simulink model "MPU9250"  (R2020b)
settings: Solver=FixedStepAuto  StartTime=0.0  StopTime=inf  FixedStep=1/500  RelTol=1e-3
libraries: sm_lib x4, nesl_utility x4, mspfiltlib x1, arduinosensorlib x1
settings Model: SILPILModeSetting=veronly  ExtModeTrigDuration=2  Creator=Tommaso  LastModifiedBy=Tommaso
settings OptimizationCC: EnhancedBackFolding=on  PassReuseOutputArgsAs=Individual arguments  ZeroExternalMemoryAtStartup=off  ZeroInternalMemoryAtStartup=off  MaxStackSize=64  OptimizeBlockOrder=speed  DifferentSizesBufferReuse=on  OptimizationCustomize=off  EfficientTunableParamExpr=on
settings DebuggingCC: ParameterTunabilityLossMsg=error
settings HardwareCC: ProdBitPerInt=16  ProdBitPerPointer=16  ProdBitPerSizeT=16  ProdBitPerPtrDiffT=16  ProdLargestAtomicFloat=None  ProdWordSize=8  ProdHWDeviceType=Atmel->AVR  UseEmbeddedCoderFeatures=off  UseSimulinkCoderFeatures=off
settings SFSimCC: MATLABDynamicMemAlloc=off
settings RTWCC: Description=Embedded Coder  SystemTargetFile=ert.tlc  HardwareBoard=Arduino Uno  TemplateMakefile=ert_default_tmf  Toolchain=Arduino AVR
settings CodeAppCC: ForceParamTrailComments=on  IgnoreCustomStorageClasses=off  OperatorAnnotations=on  SimulinkDataObjDesc=on  SFDataObjDesc=on  InsertBlockDesc=on
settings ERTTargetCC: SupportContinuousTime=on  SupportNonInlinedSFcns=on  SupportVariableSizeSignals=on  ExtModeStaticAllocSize=250
settings ExplorerConfigSet: InternalSimMechanicsExplorerSettings="<ExplorerConfiguration><canonicalview>aerospace</canonicalview><AnimationSetting><BasePlaybackSpeed>1.0</BasePlaybackSpeed><PlaybackSpeedFactor>1.0</PlaybackSpeedFactor></AnimationSetting><TilePanel><TileInfo><Tiles Columns=\"1\" Count=\"1\" Rows=\"1\"><Column Weight=\"1\"/><Row Weight=\"1\"/><Tile Height=\"1\" Width=\"1\" X=\"0\" Y=\"0\"/></Tiles></TileInfo><SceneInfo><SceneViewer><BGColor><R>1</R><G>1</G><B>1</B></BGColor><Camera><DoPerspective>off</DoPerspective><Position><X>-0.693082754697760484</X><Y>0.369421598530021988</Y><Z>-0.361362961081841516</Z></Position><Center><X>0.12253292156436324</X><Y>-0.0789962126630676664</Y><Z>0.00427693723400418557</Z></Center><Up><X>0.320163956155274265</X><Y>-0.176600674730688856</Y><Z>-0.930756274684016782</Z></Up><ViewLimDist>1</ViewLimDist><YLim>0.1588242526875695</YLim><XLim>0.267697134651695201</XLim></Camera></SceneViewer></SceneInfo></TilePanel><MechEditorPanel><Cameras/><GfxPanelCameraMap/><VideoCreator><PlaybackSpeedRatio>1.0</PlaybackSpeedRatio><FrameRate>30</FrameRate><VideoFormat>Motion JPEG AVI</VideoFormat><FrameSize>auto</FrameSize></VideoCreator></MechEditorPanel></ExplorerConfiguration>"

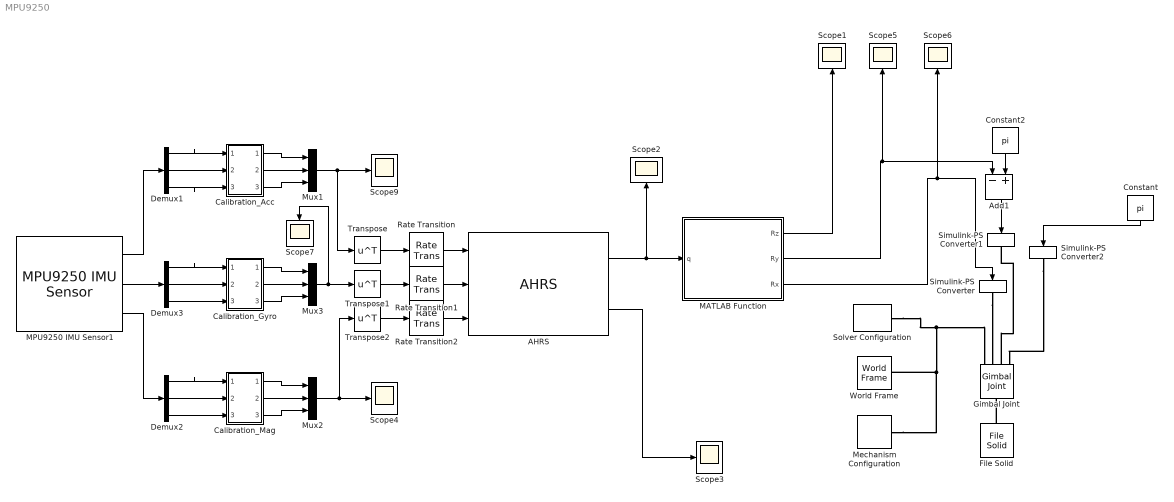
== system MPU9250 ==
  AHRS : mspfiltlib/AHRS  DispRefFrame=NED  DecimationFactor=1  InitialProcessNoise=ahrsfilter.defaultProcessNoise  OrientationFormat=quaternion  SimulateUsing=Interpreted execution  AccelerometerNoise=0.05  GyroscopeNoise=1  MagnetometerNoise=3  GyroscopeDriftNoise=3.0462e-3  LinearAccelerationNoise=0.01  MagneticDisturbanceNoise=0.5  LinearAccelerationDecayFactor=0.14  MagneticDisturbanceDecayFactor=0.08  ExpectedMagneticFieldStrength=40
      settings: SourceProductBaseCode=TF,NV
  Add1 : Sum  Inputs=-+
  Calibration_Acc : Subsystem
  Calibration_Gyro : Subsystem
  Calibration_Mag : Subsystem
  Constant : Constant  Value=pi
  Constant2 : Constant  Value=pi
  Demux1 : Demux  Outputs=3
  Demux2 : Demux  Outputs=3
  Demux3 : Demux  Outputs=3
  File Solid : sm_lib/Body Elements/File Solid  ExtGeomFileName=C:\Users\Tommaso\università\Controlli Automatici\Progetto\Solidworks\Drone.stl  UnitType=Custom  ExtGeomFileUnits=mm  StepReaderType=HEX  ExportConvexHullGeometry=off  InertiaType=Custom  Mass=1  MassUnits=kg  CenterOfMass=[150 150 40]  CenterOfMassUnits=mm  MomentsOfInertia=[1 1 1]  MomentsOfInertiaUnits=kg*m^2  ProductsOfInertia=[0 0 0]  ProductsOfInertiaUnits=kg*m^2  BasedOnType=DensityFromFile  Density=1000  DensityUnits=kg/m^3  DoExposeReferenceFrame=off  SerializedFrames=<Frames><Frame><Id>Frame1</Id><Value><Name>F1</Name><Origin><Source>CenterOfMassFrame</Source><FeatureName></FeatureName></Origin><PrimaryAxis><DefinedDirection>+Z</DefinedDirection><Source>ReferenceFrame</Source><SourceDirection>-Z</SourceDirection><FeatureName></FeatureName></PrimaryAxis><SecondaryAxis><DefinedDirection>+X</DefinedDirection><Source>ReferenceFrame</Source><SourceDirection>-X</SourceDirection><FeatureName></FeatureName></SecondaryAxis></Value></Frame></Frames>  GraphicType=FromGeometry  MarkerShape=Sphere  MarkerSize=10  GraphicVisPropType=SimpleVisualProperties  GraphicDiffuseColor=[0.6 0.6 0.6]  GraphicSpecularColor=[0.5 0.5 0.5 1.0]  GraphicAmbientColor=[0.15 0.15 0.15 1.0]  GraphicEmissiveColor=[0.0 0.0 0.0 1.0]  GraphicShininess=75  GraphicOpacity=1.0
  Gimbal Joint : sm_lib/Joints/Gimbal Joint  JointMode=Normal  SenseConstraintForce=off  SenseConstraintForceX=off  SenseConstraintForceY=off  SenseConstraintForceZ=off  SenseConstraintTorque=off  SenseConstraintTorqueX=off  SenseConstraintTorqueY=off  SenseConstraintTorqueZ=off  SenseTotalForce=off  SenseTotalForceX=off  SenseTotalForceY=off  SenseTotalForceZ=off  SenseTotalTorque=off  SenseTotalTorqueX=off  SenseTotalTorqueY=off  SenseTotalTorqueZ=off  CompositeWrenchDir=FollowerOnBase  CompositeWrenchFrame=BaseFrame  RxEquilibriumPosition=0  RxEquilibriumPositionUnits=deg  RxSpringStiffness=0  RxSpringStiffnessUnits=N*m/deg  RxDampingCoefficient=0  RxDampingCoefficientUnits=N*m/(deg/s)  RxTorqueActuationMode=ComputedTorque  RxMotionActuationMode=InputMotion  RxSensePosition=off  RxSenseVelocity=off  RxSenseAcceleration=off  RxSenseTorqueForce=off  RxSenseLowerLimitTorqueForce=off  RxSenseUpperLimitTorqueForce=off  RxLowerLimitSpecify=off  RxLowerLimitBound=-90  RxLowerLimitBoundUnits=deg  RxLowerLimitStiffness=1e4  RxLowerLimitStiffnessUnits=N*m/deg  RxLowerLimitDamping=10  RxLowerLimitDampingUnits=N*m/(deg/s)  RxLowerLimitTransitionRegionWidth=0.1  RxLowerLimitTransitionRegionWidthUnits=deg  RxUpperLimitSpecify=off  RxUpperLimitBound=90  RxUpperLimitBoundUnits=deg  RxUpperLimitStiffness=1e4  RxUpperLimitStiffnessUnits=N*m/deg  RxUpperLimitDamping=10  RxUpperLimitDampingUnits=N*m/(deg/s)  RxUpperLimitTransitionRegionWidth=0.1  RxUpperLimitTransitionRegionWidthUnits=deg  RxPositionTargetSpecify=off  RxPositionTargetPriority=High  RxPositionTargetValue=0  RxPositionTargetValueUnits=deg  RxVelocityTargetSpecify=off  RxVelocityTargetPriority=High  RxVelocityTargetValue=0  RxVelocityTargetValueUnits=deg/s  RyEquilibriumPosition=0  RyEquilibriumPositionUnits=deg  RySpringStiffness=0  RySpringStiffnessUnits=N*m/deg  RyDampingCoefficient=0  RyDampingCoefficientUnits=N*m/(deg/s)  RyTorqueActuationMode=ComputedTorque  RyMotionActuationMode=InputMotion  RySensePosition=off  RySenseVelocity=off  RySenseAcceleration=off  RySenseTorqueForce=off  RySenseLowerLimitTorqueForce=off  RySenseUpperLimitTorqueForce=off  RyLowerLimitSpecify=off  RyLowerLimitBound=-90  RyLowerLimitBoundUnits=deg  RyLowerLimitStiffness=1e4  RyLowerLimitStiffnessUnits=N*m/deg  RyLowerLimitDamping=10  RyLowerLimitDampingUnits=N*m/(deg/s)  RyLowerLimitTransitionRegionWidth=0.1  RyLowerLimitTransitionRegionWidthUnits=deg  RyUpperLimitSpecify=off  RyUpperLimitBound=90  RyUpperLimitBoundUnits=deg  RyUpperLimitStiffness=1e4  RyUpperLimitStiffnessUnits=N*m/deg  RyUpperLimitDamping=10  RyUpperLimitDampingUnits=N*m/(deg/s)  RyUpperLimitTransitionRegionWidth=0.1  RyUpperLimitTransitionRegionWidthUnits=deg  RyPositionTargetSpecify=off  RyPositionTargetPriority=High  RyPositionTargetValue=0  RyPositionTargetValueUnits=deg  RyVelocityTargetSpecify=off  RyVelocityTargetPriority=High  RyVelocityTargetValue=0  RyVelocityTargetValueUnits=deg/s  RzEquilibriumPosition=0  RzEquilibriumPositionUnits=deg  RzSpringStiffness=0  RzSpringStiffnessUnits=N*m/deg  RzDampingCoefficient=0  RzDampingCoefficientUnits=N*m/(deg/s)  RzTorqueActuationMode=ComputedTorque  RzMotionActuationMode=InputMotion  RzSensePosition=off  RzSenseVelocity=off  RzSenseAcceleration=off  RzSenseTorqueForce=off  RzSenseLowerLimitTorqueForce=off  RzSenseUpperLimitTorqueForce=off  RzLowerLimitSpecify=off  RzLowerLimitBound=-90  RzLowerLimitBoundUnits=deg  RzLowerLimitStiffness=1e4  RzLowerLimitStiffnessUnits=N*m/deg  RzLowerLimitDamping=10  RzLowerLimitDampingUnits=N*m/(deg/s)  RzLowerLimitTransitionRegionWidth=0.1  RzLowerLimitTransitionRegionWidthUnits=deg  RzUpperLimitSpecify=off  RzUpperLimitBound=90  RzUpperLimitBoundUnits=deg  RzUpperLimitStiffness=1e4  RzUpperLimitStiffnessUnits=N*m/deg  RzUpperLimitDamping=10  RzUpperLimitDampingUnits=N*m/(deg/s)  RzUpperLimitTransitionRegionWidth=0.1  RzUpperLimitTransitionRegionWidthUnits=deg  RzPositionTargetSpecify=off  RzPositionTargetPriority=High  RzPositionTargetValue=0  RzPositionTargetValueUnits=deg  RzVelocityTargetSpecify=off  RzVelocityTargetPriority=High  RzVelocityTargetValue=0  RzVelocityTargetValueUnits=deg/s
  MATLAB Function : MATLAB Function  TreatAsAtomicUnit=on
  MPU9250 IMU Sensor1 : arduinosensorlib/MPU9250 IMU Sensor  SlaveAddress=0x68  Accel=on  AngularRate=on  Ak8963Field=on  Temperature=off  Status=off  EulerAngles=off  Quat=off  AccelRange=4G  Acceldlpf=44.8 Hz  GyroRange=250 dps  Gyrodlpf=41 Hz  DmpOdr=200 Hz  SampleTime=-1
      settings: SourceProductBaseCode=ARDUINO
  Mechanism Configuration : sm_lib/Utilities/Mechanism Configuration  UniformGravity=Constant  GravityVector=[0 0 -9.80665]  GravityVectorUnits=m/s^2  GravityUnits=m/s^2  LinearizationDelta=0.001  JointModeTransitionNonlinearIterations=2
  Mux1 : Mux  Inputs=3
  Mux2 : Mux  Inputs=3
  Mux3 : Mux  Inputs=3
  Rate Transition : RateTransition
  Rate Transition1 : RateTransition
  Rate Transition2 : RateTransition
  Scope{1..7,9} (8 alike) : Scope
  Simulink-PS Converter : nesl_utility/Simulink-PS Converter  PhysicalDomain=network_engine_domain  SubClassName=ps_input  LeftPortType=input  RightPortType=output  PseudoPeriodic=off  Frequencies=[]  NoiseDistribution=none  NoiseParameters=[]  Unit=rad  AffineConversion=off  FilteringAndDerivatives=zero  SimscapeFilterOrder=1  InputFilterTimeConstant=0.001  UdotUserProvided=0
  Simulink-PS Converter1 : nesl_utility/Simulink-PS Converter  PhysicalDomain=network_engine_domain  SubClassName=ps_input  LeftPortType=input  RightPortType=output  PseudoPeriodic=off  Frequencies=[]  NoiseDistribution=none  NoiseParameters=[]  Unit=rad  AffineConversion=off  FilteringAndDerivatives=zero  SimscapeFilterOrder=1  InputFilterTimeConstant=0.001  UdotUserProvided=0
  Simulink-PS Converter2 : nesl_utility/Simulink-PS Converter  PhysicalDomain=network_engine_domain  SubClassName=ps_input  LeftPortType=input  RightPortType=output  PseudoPeriodic=off  Frequencies=[]  NoiseDistribution=none  NoiseParameters=[]  Unit=rad  AffineConversion=off  FilteringAndDerivatives=zero  SimscapeFilterOrder=1  InputFilterTimeConstant=0.001  UdotUserProvided=0
  Solver Configuration : nesl_utility/Solver Configuration  PhysicalDomain=network_engine_domain  SubClassName=solver  LeftPortType=input  RightPortType=generic  Tones=[]  Harmonics=[]  SimulateNoise=off  Profile=off  UseLocalSampling=off  EnableSwitchedLinearOptims=on  FrequencyDomain=off  UseCCode=off  RelTol=0.001  AbsTol=1e-06  MinStep=1e-09  ToWorkspace=off  RevertToSquareIcSolve=off  NumHomotopyIterations=100  PhasorMode=off  PhasorModeNumHarmonics=1  DoDC=off  ResidualTolerance=1e-09  UseLocalSolver=off  LocalSolverChoice=NE_BACKWARD_EULER_ADVANCER  LocalSolverSampleTime=0.001  DoFixedCost=off  MaxNonlinIter=3  MaxModeIter=2  ComputeImpulses=off  ImpulseIterations=2  LinearAlgebra=auto  EquationFormulation=NE_TIME_EF  DelaysMemoryBudget=1024  AutomaticFiltering=on  FilteringTimeConstant=0.001  PartitionStorageMethod=AS_NEEDED  PartitionMemoryBudget=1024  PartitionMethod=ROBUST
  Transpose : Math  Operator=transpose  SaturateOnIntegerOverflow=on
  Transpose1 : Math  Operator=transpose  SaturateOnIntegerOverflow=on
  Transpose2 : Math  Operator=transpose  SaturateOnIntegerOverflow=on
  World Frame : sm_lib/Frames and Transforms/World Frame
  wires:
  MPU9250 IMU Sensor1/1 -> Demux1/1
  Demux1/1 -> Calibration_Acc/1(In1)
  Demux1/2 -> Calibration_Acc/2(In2)
  Demux1/3 -> Calibration_Acc/3(In3)
  Calibration_Acc/1(Out1) -> Mux1/1
  Calibration_Acc/2(Out2) -> Mux1/2
  Calibration_Acc/3(Out3) -> Mux1/3
  Mux1/1 -> Scope9/1, Transpose/1
  MPU9250 IMU Sensor1/2 -> Demux3/1
  Transpose/1 -> Rate Transition/1
  Transpose1/1 -> Rate Transition1/1
  Transpose2/1 -> Rate Transition2/1
  AHRS/1 -> Scope2/1, MATLAB Function/1(q)
  AHRS/2 -> Scope3/1
  Mux2/1 -> Scope4/1, Transpose2/1
  Calibration_Mag/2(Out2) -> Mux2/2
  Demux2/2 -> Calibration_Mag/2(In2)
  Calibration_Mag/1(Out1) -> Mux2/1
  Demux2/1 -> Calibration_Mag/1(In1)
  MPU9250 IMU Sensor1/3 -> Demux2/1
  Calibration_Mag/3(Out3) -> Mux2/3
  Demux2/3 -> Calibration_Mag/3(In3)
  Rate Transition2/1 -> AHRS/3
  Rate Transition1/1 -> AHRS/2
  Rate Transition/1 -> AHRS/1
  Demux3/2 -> Calibration_Gyro/2(In2)
  Demux3/3 -> Calibration_Gyro/3(In3)
  Calibration_Gyro/2(Out2) -> Mux3/2
  Demux3/1 -> Calibration_Gyro/1(In1)
  Calibration_Gyro/3(Out3) -> Mux3/3
  Calibration_Gyro/1(Out1) -> Mux3/1
  Mux3/1 -> Transpose1/1, Scope7/1
  MATLAB Function/1(Rz) -> Scope1/1
  MATLAB Function/2(Ry) -> Add1/1, Scope5/1
  MATLAB Function/3(Rx) -> Simulink-PS Converter/1, Scope6/1
  Add1/1 -> Simulink-PS Converter1/1
  Constant2/1 -> Add1/2
  Constant/1 -> Simulink-PS Converter2/1
  connections:
  World Frame/RConn1 -- Solver Configuration/RConn1 -- Gimbal Joint/LConn1 -- Mechanism Configuration/RConn1
  File Solid/LConn1 -- Gimbal Joint/RConn1
  Simulink-PS Converter2/RConn1 -- Gimbal Joint/LConn4
  Gimbal Joint/LConn3 -- Simulink-PS Converter1/RConn1
  Simulink-PS Converter/RConn1 -- Gimbal Joint/LConn2

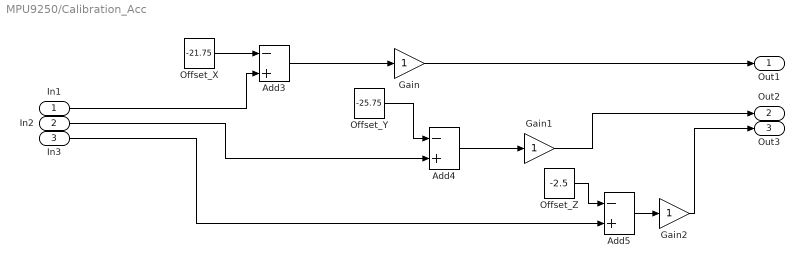
== system MPU9250/Calibration_Acc ==
  In1 : Inport
  In2 : Inport  Port=2
  In3 : Inport  Port=3
  Add3 : Sum  Inputs=-+
  Add4 : Sum  Inputs=-+
  Add5 : Sum  Inputs=-+
  Gain : Gain
  Gain1 : Gain
  Gain2 : Gain
  Offset_X : Constant  Value=-21.75
  Offset_Y : Constant  Value=-25.75
  Offset_Z : Constant  Value=-2.5
  Out1 : Outport
  Out2 : Outport  Port=2
  Out3 : Outport  Port=3
  wires:
  Offset_Y/1 -> Add4/1
  In2/1 -> Add4/2
  Add5/1 -> Gain2/1
  Offset_X/1 -> Add3/1
  Offset_Z/1 -> Add5/1
  In3/1 -> Add5/2
  Add4/1 -> Gain1/1
  In1/1 -> Add3/2
  Add3/1 -> Gain/1
  Gain2/1 -> Out3/1
  Gain1/1 -> Out2/1
  Gain/1 -> Out1/1

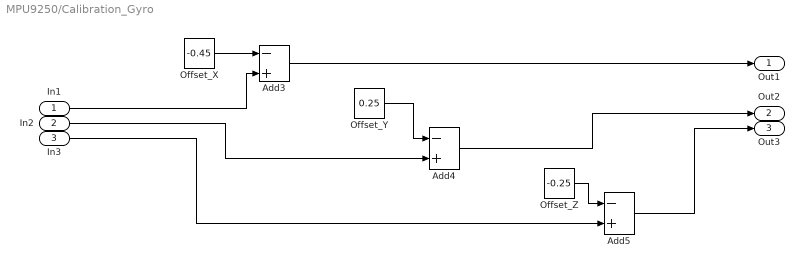
== system MPU9250/Calibration_Gyro ==
  In1 : Inport
  In2 : Inport  Port=2
  In3 : Inport  Port=3
  Add3 : Sum  Inputs=-+
  Add4 : Sum  Inputs=-+
  Add5 : Sum  Inputs=-+
  Offset_X : Constant  Value=-0.45
  Offset_Y : Constant  Value=0.25
  Offset_Z : Constant  Value=-0.25
  Out1 : Outport
  Out2 : Outport  Port=2
  Out3 : Outport  Port=3
  wires:
  Offset_Y/1 -> Add4/1
  In2/1 -> Add4/2
  Offset_X/1 -> Add3/1
  Offset_Z/1 -> Add5/1
  In3/1 -> Add5/2
  In1/1 -> Add3/2
  Add5/1 -> Out3/1
  Add4/1 -> Out2/1
  Add3/1 -> Out1/1

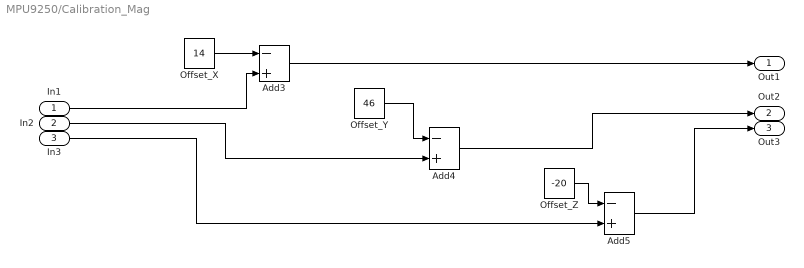
== system MPU9250/Calibration_Mag ==
  In1 : Inport
  In2 : Inport  Port=2
  In3 : Inport  Port=3
  Add3 : Sum  Inputs=-+
  Add4 : Sum  Inputs=-+
  Add5 : Sum  Inputs=-+
  Offset_X : Constant  Value=14
  Offset_Y : Constant  Value=46
  Offset_Z : Constant  Value=-20
  Out1 : Outport
  Out2 : Outport  Port=2
  Out3 : Outport  Port=3
  wires:
  Offset_Y/1 -> Add4/1
  In2/1 -> Add4/2
  Offset_X/1 -> Add3/1
  Offset_Z/1 -> Add5/1
  In3/1 -> Add5/2
  In1/1 -> Add3/2
  Add5/1 -> Out3/1
  Add4/1 -> Out2/1
  Add3/1 -> Out1/1

== matlab function MPU9250/MATLAB Function ==
  data: q input; Rz output; Ry output; Rx output
function [Rz, Ry, Rx] = quattoangle(q)
q0 = q(1);
q1 = q(2);
q2 = q(3);
q3 = q(4);

Rx =  atan(2*(q2*q3+q0*q1)/(q0^2-q1^2-q2^2+q3^2));
Ry =  asin(-2*(q1*q3-q0*q2));
Rz =  atan(2*(q1*q2+q0*q3)/(q0^2+q1^2-q2^2-q3^2));
end
